simulink model "LLA_to_ECEF"  (R2022a)
settings: Solver=VariableStepAuto  StartTime=0.0  StopTime=1739  RelTol=1e-3
values from neighbouring files (symbols this model uses):
  fs = 1/3    (= 0.333333333333)    [p2.m]
settings Model: Creator=jorch  LastModifiedBy=jorch

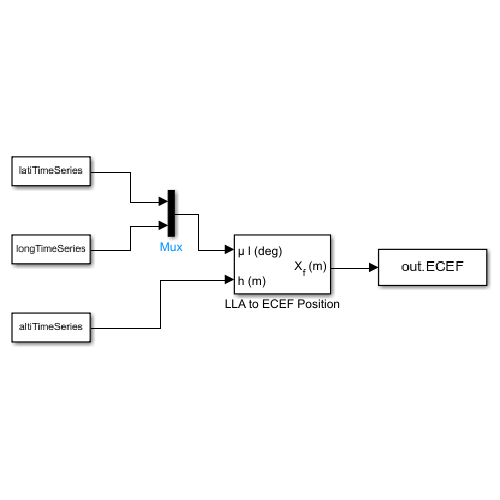
[thumbnail: Simulink's stored preview of the top-level diagram]
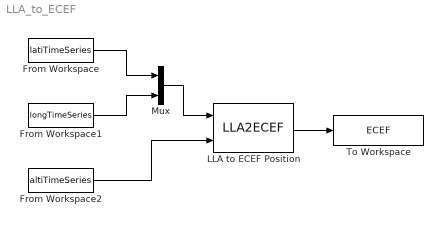
== system LLA_to_ECEF ==
  From Workspace : FromWorkspace  VariableName=latiTimeSeries  SampleTime=fs
  From Workspace1 : FromWorkspace  VariableName=longTimeSeries  SampleTime=fs
  From Workspace2 : FromWorkspace  VariableName=altiTimeSeries  SampleTime=fs
  LLA to ECEF Position : LLA2ECEF
  Mux : Mux  Inputs=2
  To Workspace : ToWorkspace  VariableName=ECEF  SampleTime=fs
  wires:
  From Workspace/1 -> Mux/1
  From Workspace1/1 -> Mux/2
  Mux/1 -> LLA to ECEF Position/1
  From Workspace2/1 -> LLA to ECEF Position/2
  LLA to ECEF Position/1 -> To Workspace/1
